simulink model "two_area_bus_system"  (R2023b)
settings: Solver=VariableStepAuto  StartTime=0.0  StopTime=20  RelTol=1e-3
libraries: eeGeneralControl x1
settings Model: Creator=Sandeep  LastModifiedBy=LENOVO
settings DataIOCC: ReturnWorkspaceOutputs=off
settings ModelReferenceCC: EnableRefExpFcnMdlSchedulingChecks=on

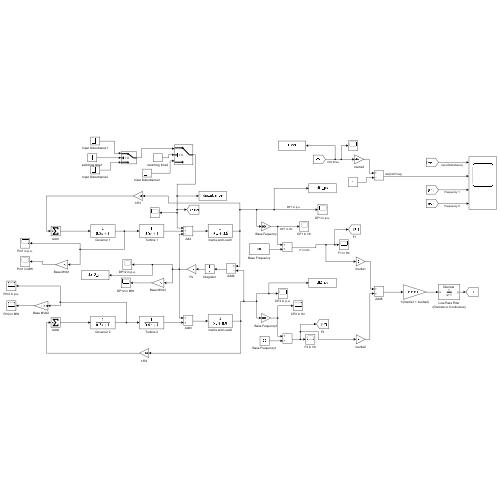
[thumbnail: Simulink's stored preview of the top-level diagram]
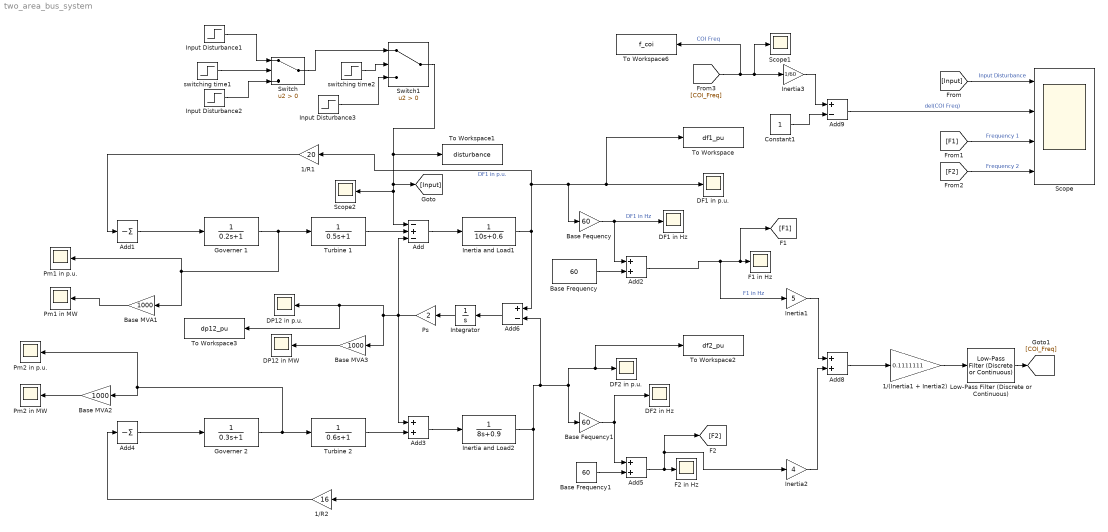
== system two_area_bus_system ==
  1/(Inertia1 + Inertia2) : Gain  Gain=0.1111111
  1/R1 : Gain  Gain=20
  1/R2 : Gain  Gain=16
  Add : Sum  Inputs=-+-
  Add1 : Sum  Inputs=-
  Add{2..3,5,8} (4 alike) : Sum
  Add4 : Sum  Inputs=-
  Add6 : Sum  Inputs=+-
  Add9 : Sum  Inputs=+-
  Base Fequency : Gain  Gain=60
  Base Fequency1 : Gain  Gain=60
  Base Frequency : Constant  Value=60
  Base Frequency1 : Constant  Value=60
  Base MVA1 : Gain  Gain=1000
  Base MVA2 : Gain  Gain=1000
  Base MVA3 : Gain  Gain=1000
  Constant1 : Constant
  DF1 in Hz : Scope
  DF1 in p.u. : Scope
  DF2 in Hz : Scope
  DF2 in p.u. : Scope
  DP12 in MW : Scope
  DP12 in p.u. : Scope
  F1 in Hz : Scope
  F2 in Hz : Scope
  Governer 1 : TransferFcn  Denominator=[0.2,1]
  Governer 2 : TransferFcn  Denominator=[0.3,1]
  Inertia and Load1 : TransferFcn  Denominator=[10 0.6]
  Inertia and Load2 : TransferFcn  Denominator=[8 0.9]
  Inertia1 : Gain  Gain=5
  Inertia2 : Gain  Gain=4
  Inertia3 : Gain  Gain=1/60
  Input Disturbance1 : Step  Time=0  After=0  SampleTime=0
  Input Disturbance2 : Step  Time=2.5  SampleTime=0
  Input Disturbance3 : Step  Time=3  After=0  SampleTime=0
  Integrator : Integrator
  Low-Pass Filter (Discrete or Continuous) : eeGeneralControl/Low-Pass Filter (Discrete or Continuous)  K=1  T=1  B=inf  A=-inf  init_option=Inherited from block input  x0=0  Ts=-1
  Pm1 in MW : Scope
  Pm1 in p.u. : Scope
  Pm2 in MW : Scope
  Pm2 in p.u. : Scope
  Ps : Gain  Gain=2
  Scope : Scope  NumInputPorts=4
  Scope1 : Scope
  Scope2 : Scope
  Switch : Switch  Criteria=u2 > Threshold  SaturateOnIntegerOverflow=off  InputSameDT=off
  Switch1 : Switch  Criteria=u2 > Threshold  SaturateOnIntegerOverflow=off  InputSameDT=off
  To Workspace : ToWorkspace  VariableName=df1_pu  SampleTime=0.01
  To Workspace1 : ToWorkspace  VariableName=disturbance  SampleTime=-1
  To Workspace2 : ToWorkspace  VariableName=df2_pu  SampleTime=0.01
  To Workspace3 : ToWorkspace  VariableName=dp12_pu  SampleTime=0.01
  To Workspace6 : ToWorkspace  VariableName=f_coi  SampleTime=0.01
  Turbine 1 : TransferFcn  Denominator=[0.5 1]
  Turbine 2 : TransferFcn  Denominator=[0.6 1]
  switching time1 : Step  Time=2.5  Before=1  After=0  SampleTime=0
  switching time2 : Step  Time=3  Before=1  After=0  SampleTime=0
  wires:
  Turbine 1/1 -> Add/2
  Add/1 -> Inertia and Load1/1
  Governer 1/1 -> Base MVA1/1, Pm1 in p.u./1, Turbine 1/1
  Add1/1 -> Governer 1/1
  Inertia and Load1/1 -> 1/R1/1, Base Fequency/1, To Workspace/1, DF1 in p.u./1, Add6/1  "DF1 in p.u."
  1/R1/1 -> Add1/1
  Base Fequency/1 -> Add2/1, DF1 in Hz/1  "DF1 in Hz"
  Add2/1 -> Inertia1/1, [F1], F1 in Hz/1  "F1 in Hz"
  Base Frequency/1 -> Add2/2
  Base Fequency1/1 -> Add5/1, DF2 in Hz/1
  Base Frequency1/1 -> Add5/2
  Add5/1 -> [F2], Inertia2/1, F2 in Hz/1
  Inertia and Load2/1 -> 1/R2/1, Add6/2, Base Fequency1/1, To Workspace2/1, DF2 in p.u./1
  Turbine 2/1 -> Add3/2
  Add4/1 -> Governer 2/1
  1/R2/1 -> Add4/1
  Add3/1 -> Inertia and Load2/1
  Base MVA1/1 -> Pm1 in MW/1
  Base MVA2/1 -> Pm2 in MW/1
  Governer 2/1 -> Pm2 in p.u./1, Base MVA2/1, Turbine 2/1
  Add6/1 -> Integrator/1
  Integrator/1 -> Ps/1
  Base MVA3/1 -> DP12 in MW/1
  Ps/1 -> To Workspace3/1, DP12 in p.u./1, Base MVA3/1, Add/3, Add3/1
  [Input] -> Scope/1  "Input Disturbance"
  [F1] -> Scope/3  "Frequency 1"
  [F2] -> Scope/4  "Frequency 2"
  Inertia1/1 -> Add8/1
  Inertia2/1 -> Add8/2
  Add8/1 -> 1/(Inertia1 + Inertia2)/1
  Add9/1 -> Scope/2  "del(COI Freq)"
  Low-Pass Filter (Discrete or Continuous)/1 -> [COI_Freq]
  1/(Inertia1 + Inertia2)/1 -> Low-Pass Filter (Discrete or Continuous)/1
  Constant1/1 -> Add9/2
  [COI_Freq] -> To Workspace6/1, Scope1/1, Inertia3/1  "COI Freq"
  Inertia3/1 -> Add9/1
  switching time1/1 -> Switch/2
  Input Disturbance1/1 -> Switch/1
  Input Disturbance2/1 -> Switch/3
  Switch/1 -> Switch1/1
  Input Disturbance3/1 -> Switch1/3
  switching time2/1 -> Switch1/2
  Switch1/1 -> To Workspace1/1, [Input], Add/1, Scope2/1
